simulink model "gm_uz_pu_conversion"  (R2021a)
settings: Solver=FixedStepDiscrete  StartTime=0.0  StopTime=0.02  RelTol=1e-3
undefined symbols (not defined in the file or in its folder): ampl, freq_Hz, I_B, t_ADC, V_B, v_dc
libraries: spsThreePhaseSineGeneratorLib x3
settings Model: Creator=micha  LastModifiedBy=micha
settings SolverCC: AlgebraicLoopSolver=TrustRegion
settings DataIOCC: LimitDataPoints=on  SaveOutput=off  SaveTime=off
settings OptimizationCC: BlockReduction=off  ConditionallyExecuteInputs=off  DefaultParameterBehavior=Inlined  LifeSpan=inf
settings DebuggingCC: AlgebraicLoopMsg=error  InheritedTsInSrcMsg=none  SingleTaskRateTransMsg=error  AllowSymbolicDim=off  StrictBusMsg=ErrorOnBusTreatedAsVector  SFUnexpectedBacktrackingDiag=warning  SFNoUnconditionalDefaultTransitionDiag=warning  SFExecutionAtInitializationDiag=none  SFMachineParentedDataDiag=warning  ArithmeticOperatorsInVariantConditions=warning
settings HardwareCC: ProdBitPerPointer=32  ProdBitPerSizeT=32  ProdBitPerPtrDiffT=32  ProdLargestAtomicFloat=None  ProdIntDivRoundTo=Undefined  ProdEndianess=Unspecified  ProdWordSize=32  ProdHWDeviceType=ASIC/FPGA->ASIC/FPGA  ProdEqTarget=off
settings SFSimCC: SimUseLocalCustomCode=off  CustomCodeUndefinedFunction=UseInterfaceOnly
settings RTWCC: RTWUseLocalCustomCode=off
settings CodeAppCC: StateflowObjectComments=on
settings GRTTargetCC: TargetLangStandard=C89/C90 (ANSI)
settings ConfigComp: CovScope=ReferencedModels  CovMetricSettings=dw  CovSaveCumulativeToWorkspaceVar=on  CovSaveSingleToWorkspaceVar=on  CovExternalEMLEnable=off  CovSFcnEnable=off

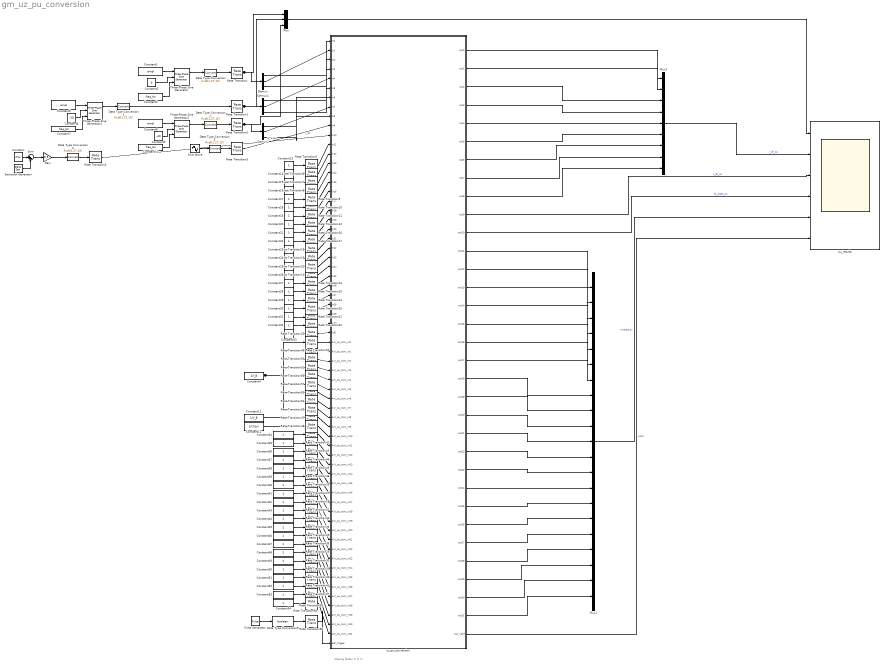
== system gm_uz_pu_conversion ==
  note: sharing factor = 0 !!!
  Constant : Constant  Value=2*pi
  Constant1 : Constant  Value=ampl
  Constant10 : Constant  Value=freq_Hz
  Constant11 : Constant  Value=1/V_B  OutDataTypeStr=fixdt(0,18,18)
  Constant12 : Constant  Value=1/(2*pi)  OutDataTypeStr=fixdt(0,18,18)
  Constant{13..33} (21 alike) : Constant  OutDataTypeStr=fixdt(1,27,15)
  Constant2 : Constant  Value=0
  Constant3 : Constant  Value=freq_Hz
  Constant{34..54} (21 alike) : Constant  OutDataTypeStr=fixdt(0,18,18)
  Constant4 : Constant  Value=1/I_B  OutDataTypeStr=fixdt(0,18,18)
  Constant5 : Constant  Value=ampl
  Constant6 : Constant  Value=-20
  Constant7 : Constant  Value=freq_Hz
  Constant8 : Constant  Value=ampl
  Constant9 : Constant  Value=-40
  Data Type Conversion{,1..4} (5 alike) : DataTypeConversion  OutDataTypeStr=fixdt(1,27,15)
  Data Type Conversion5 : DataTypeConversion  OutDataTypeStr=boolean
  Demux : Demux  Outputs=3
  Demux1 : Demux  Outputs=3
  Demux2 : Demux  Outputs=3
  Gain : Gain  Gain=0.5
  Mux : Mux  Inputs=3
  Mux1 : Mux  Inputs=21
  Mux3 : Mux  Inputs=9
  Pulse Generator : DiscretePulseGenerator  PulseType=Time based  Period=t_ADC  PulseWidth=5
  Rate Transition{,1..58} (59 alike) : RateTransition  OutPortSampleTime=ts
  Sawtooth Generator : SignalGenerator  WaveForm=sawtooth  Amplitude=2*pi  Frequency=2*pi*freq_Hz  Units=rad/sec
  Sine Wave : Sin  Amplitude=0.03*v_dc  Bias=v_dc  Frequency=2*pi*2*9*freq_Hz  SampleTime=0
  Sum : Sum  Inputs=|+-
  Three-Phase Sine Generator : spsThreePhaseSineGeneratorLib/Three-Phase Sine Generator  Ts=10e-9
      settings: SourceProductBaseCode=PS
  Three-Phase Sine Generator1 : spsThreePhaseSineGeneratorLib/Three-Phase Sine Generator  Ts=10e-9
      settings: SourceProductBaseCode=PS
  Three-Phase Sine Generator2 : spsThreePhaseSineGeneratorLib/Three-Phase Sine Generator  Ts=10e-9
      settings: SourceProductBaseCode=PS
  pu_results : Scope  NumInputPorts=6
  uz_pu_conversion : Subsystem  TreatAsAtomicUnit=on
  wires:
  uz_pu_conversion/33(out_valid) -> pu_results/6  "valid"
  Rate Transition58/1 -> uz_pu_conversion/65(adc_trigger)
  Pulse Generator/1 -> Data Type Conversion5/1
  Data Type Conversion5/1 -> Rate Transition58/1
  Mux1/1 -> pu_results/5  "unused_pu"
  uz_pu_conversion/32(out31) -> Mux1/21
  uz_pu_conversion/31(out30) -> Mux1/20
  uz_pu_conversion/30(out29) -> Mux1/19
  uz_pu_conversion/29(out28) -> Mux1/18
  uz_pu_conversion/28(out27) -> Mux1/17
  uz_pu_conversion/27(out26) -> Mux1/16
  uz_pu_conversion/26(out25) -> Mux1/15
  uz_pu_conversion/25(out24) -> Mux1/14
  uz_pu_conversion/24(out23) -> Mux1/13
  uz_pu_conversion/23(out22) -> Mux1/12
  uz_pu_conversion/22(out21) -> Mux1/11
  uz_pu_conversion/21(out20) -> Mux1/10
  uz_pu_conversion/20(out19) -> Mux1/9
  uz_pu_conversion/19(out18) -> Mux1/8
  uz_pu_conversion/18(out17) -> Mux1/7
  uz_pu_conversion/17(out16) -> Mux1/6
  uz_pu_conversion/16(out15) -> Mux1/5
  uz_pu_conversion/15(out14) -> Mux1/4
  uz_pu_conversion/14(out13) -> Mux1/3
  uz_pu_conversion/13(out12) -> Mux1/2
  uz_pu_conversion/12(out11) -> Mux1/1
  Constant52/1 -> Rate Transition37/1
  Constant51/1 -> Rate Transition41/1
  Constant50/1 -> Rate Transition40/1
  Constant54/1 -> Rate Transition39/1
  Constant53/1 -> Rate Transition38/1
  Constant42/1 -> Rate Transition32/1
  Constant43/1 -> Rate Transition33/1
  Constant44/1 -> Rate Transition34/1
  Constant48/1 -> Rate Transition30/1
  Constant45/1 -> Rate Transition35/1
  Constant49/1 -> Rate Transition31/1
  Constant46/1 -> Rate Transition36/1
  Constant47/1 -> Rate Transition29/1
  Constant38/1 -> Rate Transition46/1
  Constant39/1 -> Rate Transition26/1
  Constant40/1 -> Rate Transition27/1
  Constant41/1 -> Rate Transition28/1
  Constant36/1 -> Rate Transition44/1
  Constant37/1 -> Rate Transition45/1
  Constant35/1 -> Rate Transition43/1
  Constant34/1 -> Rate Transition42/1
  Constant33/1 -> Rate Transition23/1
  Constant31/1 -> Rate Transition21/1
  Constant32/1 -> Rate Transition22/1
  Constant29/1 -> Rate Transition24/1
  Constant30/1 -> Rate Transition25/1
  Constant28/1 -> Rate Transition15/1
  Constant27/1 -> Rate Transition14/1
  Constant25/1 -> Rate Transition20/1
  Constant26/1 -> Rate Transition13/1
  Constant24/1 -> Rate Transition19/1
  Constant23/1 -> Rate Transition18/1
  Constant21/1 -> Rate Transition16/1
  Constant22/1 -> Rate Transition17/1
  Constant20/1 -> Rate Transition12/1
  Constant19/1 -> Rate Transition11/1
  Constant17/1 -> Rate Transition9/1
  Constant18/1 -> Rate Transition10/1
  Constant16/1 -> Rate Transition8/1
  Constant15/1 -> Rate Transition7/1
  Constant14/1 -> Rate Transition6/1
  Constant13/1 -> Rate Transition5/1
  Rate Transition1/1 -> Demux1/1, Mux/2
  Mux/1 -> pu_results/1
  Rate Transition56/1 -> uz_pu_conversion/37(AXI_pu_conv_in4)
  Rate Transition57/1 -> uz_pu_conversion/38(AXI_pu_conv_in5)
  Rate Transition55/1 -> uz_pu_conversion/41(AXI_pu_conv_in8)
  Rate Transition54/1 -> uz_pu_conversion/40(AXI_pu_conv_in7)
  Rate Transition51/1 -> uz_pu_conversion/36(AXI_pu_conv_in3)
  Rate Transition52/1 -> uz_pu_conversion/33(AXI_pu_conv_in0)
  Rate Transition53/1 -> uz_pu_conversion/39(AXI_pu_conv_in6)
  Rate Transition49/1 -> uz_pu_conversion/34(AXI_pu_conv_in1)
  Rate Transition50/1 -> uz_pu_conversion/35(AXI_pu_conv_in2)
  Rate Transition48/1 -> uz_pu_conversion/43(AXI_pu_conv_in10)
  Rate Transition47/1 -> uz_pu_conversion/42(AXI_pu_conv_in9)
  Rate Transition42/1 -> uz_pu_conversion/44(AXI_pu_conv_in11)
  Rate Transition33/1 -> uz_pu_conversion/53(AXI_pu_conv_in20)
  Rate Transition29/1 -> uz_pu_conversion/57(AXI_pu_conv_in24)
  Rate Transition46/1 -> uz_pu_conversion/48(AXI_pu_conv_in15)
  Rate Transition35/1 -> uz_pu_conversion/55(AXI_pu_conv_in22)
  Rate Transition28/1 -> uz_pu_conversion/51(AXI_pu_conv_in18)
  Rate Transition44/1 -> uz_pu_conversion/46(AXI_pu_conv_in13)
  Rate Transition45/1 -> uz_pu_conversion/47(AXI_pu_conv_in14)
  Rate Transition40/1 -> uz_pu_conversion/60(AXI_pu_conv_in27)
  Rate Transition26/1 -> uz_pu_conversion/49(AXI_pu_conv_in16)
  Rate Transition27/1 -> uz_pu_conversion/50(AXI_pu_conv_in17)
  Rate Transition37/1 -> uz_pu_conversion/62(AXI_pu_conv_in29)
  Rate Transition30/1 -> uz_pu_conversion/58(AXI_pu_conv_in25)
  Rate Transition38/1 -> uz_pu_conversion/63(AXI_pu_conv_in30)
  Rate Transition41/1 -> uz_pu_conversion/61(AXI_pu_conv_in28)
  Rate Transition39/1 -> uz_pu_conversion/64(AXI_pu_conv_in31)
  Rate Transition43/1 -> uz_pu_conversion/45(AXI_pu_conv_in12)
  Rate Transition31/1 -> uz_pu_conversion/59(AXI_pu_conv_in26)
  Rate Transition36/1 -> uz_pu_conversion/56(AXI_pu_conv_in23)
  Rate Transition32/1 -> uz_pu_conversion/52(AXI_pu_conv_in19)
  Rate Transition34/1 -> uz_pu_conversion/54(AXI_pu_conv_in21)
  Rate Transition21/1 -> uz_pu_conversion/30(in29)
  Rate Transition24/1 -> uz_pu_conversion/28(in27)
  Rate Transition25/1 -> uz_pu_conversion/29(in28)
  Rate Transition22/1 -> uz_pu_conversion/31(in30)
  Rate Transition23/1 -> uz_pu_conversion/32(in31)
  Rate Transition14/1 -> uz_pu_conversion/26(in25)
  Rate Transition15/1 -> uz_pu_conversion/27(in26)
  Rate Transition20/1 -> uz_pu_conversion/24(in23)
  Rate Transition18/1 -> uz_pu_conversion/22(in21)
  Rate Transition19/1 -> uz_pu_conversion/23(in22)
  Rate Transition17/1 -> uz_pu_conversion/21(in20)
  Rate Transition16/1 -> uz_pu_conversion/20(in19)
  Rate Transition13/1 -> uz_pu_conversion/25(in24)
  Rate Transition11/1 -> uz_pu_conversion/18(in17)
  Rate Transition12/1 -> uz_pu_conversion/19(in18)
  Rate Transition10/1 -> uz_pu_conversion/17(in16)
  Rate Transition9/1 -> uz_pu_conversion/16(in15)
  Rate Transition8/1 -> uz_pu_conversion/15(in14)
  Rate Transition7/1 -> uz_pu_conversion/14(in13)
  Rate Transition6/1 -> uz_pu_conversion/13(in12)
  Rate Transition5/1 -> uz_pu_conversion/12(in11)
  Sum/1 -> Gain/1
  Gain/1 -> Data Type Conversion4/1
  Constant/1 -> Sum/1
  uz_pu_conversion/11(out10) -> pu_results/4  "el_angle_pu"
  Constant12/1 -> Rate Transition48/1
  Sawtooth Generator/1 -> Sum/2
  Rate Transition4/1 -> uz_pu_conversion/11(in10)  "el_angle"
  Data Type Conversion4/1 -> Rate Transition4/1
  Data Type Conversion3/1 -> Rate Transition3/1
  uz_pu_conversion/10(out9) -> pu_results/3  "v_dc_pu"
  Sine Wave/1 -> Data Type Conversion3/1
  Rate Transition3/1 -> uz_pu_conversion/10(in9)  "v_dc"
  Constant11/1 -> Rate Transition47/1
  uz_pu_conversion/9(out8) -> Mux3/9
  uz_pu_conversion/8(out7) -> Mux3/8
  uz_pu_conversion/7(out6) -> Mux3/7
  Demux2/3 -> uz_pu_conversion/9(in8)
  Demux2/2 -> uz_pu_conversion/8(in7)
  Demux2/1 -> uz_pu_conversion/7(in6)
  Rate Transition2/1 -> Demux2/1, Mux/3
  Constant10/1 -> Three-Phase Sine Generator2/3
  Constant9/1 -> Three-Phase Sine Generator2/2
  Three-Phase Sine Generator2/1 -> Data Type Conversion2/1
  Constant8/1 -> Three-Phase Sine Generator2/1
  Data Type Conversion2/1 -> Rate Transition2/1
  Demux1/3 -> uz_pu_conversion/6(in5)
  Demux1/2 -> uz_pu_conversion/5(in4)
  Demux1/1 -> uz_pu_conversion/4(in3)
  Mux3/1 -> pu_results/2  "i_ph_pu"
  uz_pu_conversion/4(out3) -> Mux3/4
  uz_pu_conversion/3(out2) -> Mux3/3
  uz_pu_conversion/2(out1) -> Mux3/2
  uz_pu_conversion/1(out0) -> Mux3/1
  uz_pu_conversion/5(out4) -> Mux3/5
  uz_pu_conversion/6(out5) -> Mux3/6
  Constant4/1 -> Rate Transition55/1, Rate Transition54/1, Rate Transition53/1, Rate Transition57/1, Rate Transition51/1, Rate Transition50/1, Rate Transition49/1, Rate Transition52/1, Rate Transition56/1
  Three-Phase Sine Generator1/1 -> Data Type Conversion1/1
  Constant5/1 -> Three-Phase Sine Generator1/1
  Data Type Conversion1/1 -> Rate Transition1/1
  Constant7/1 -> Three-Phase Sine Generator1/3
  Constant6/1 -> Three-Phase Sine Generator1/2
  Demux/3 -> uz_pu_conversion/3(in2)
  Demux/2 -> uz_pu_conversion/2(in1)
  Data Type Conversion/1 -> Rate Transition/1
  Demux/1 -> uz_pu_conversion/1(in0)
  Rate Transition/1 -> Mux/1, Demux/1
  Constant3/1 -> Three-Phase Sine Generator/3
  Constant2/1 -> Three-Phase Sine Generator/2
  Constant1/1 -> Three-Phase Sine Generator/1
  Three-Phase Sine Generator/1 -> Data Type Conversion/1

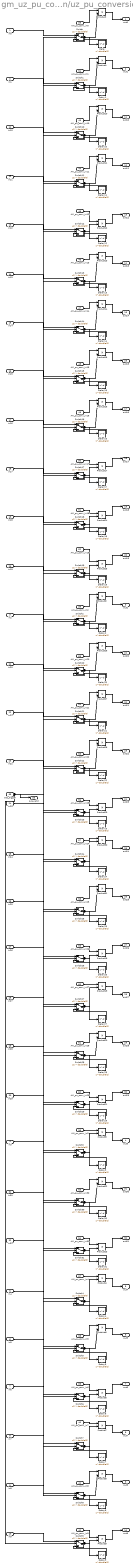
== system gm_uz_pu_conversion/uz_pu_conversion ==
  in0 : Inport  OutDataTypeStr=fixdt(1, 27, 15)  PortDimensions=1  SampleTime=1e-08
  in1 : Inport  Port=2  OutDataTypeStr=fixdt(1, 27, 15)  PortDimensions=1  SampleTime=1e-08
  in2 : Inport  Port=3  OutDataTypeStr=fixdt(1, 27, 15)  PortDimensions=1  SampleTime=1e-08
  in3 : Inport  Port=4  OutDataTypeStr=fixdt(1, 27, 15)  PortDimensions=1  SampleTime=1e-08
  in4 : Inport  Port=5  OutDataTypeStr=fixdt(1, 27, 15)  PortDimensions=1  SampleTime=1e-08
  in5 : Inport  Port=6  OutDataTypeStr=fixdt(1, 27, 15)  PortDimensions=1  SampleTime=1e-08
  in6 : Inport  Port=7  OutDataTypeStr=fixdt(1, 27, 15)  PortDimensions=1  SampleTime=1e-08
  in7 : Inport  Port=8  OutDataTypeStr=fixdt(1, 27, 15)  PortDimensions=1  SampleTime=1e-08
  in8 : Inport  Port=9  OutDataTypeStr=fixdt(1, 27, 15)  PortDimensions=1  SampleTime=1e-08
  in9 : Inport  Port=10  OutDataTypeStr=fixdt(1, 27, 15)  PortDimensions=1  SampleTime=1e-08
  in10 : Inport  Port=11  OutDataTypeStr=fixdt(1, 27, 15)  PortDimensions=1  SampleTime=1e-08
  in11 : Inport  Port=12  OutDataTypeStr=fixdt(1, 27, 15)  PortDimensions=1  SampleTime=1e-08
  in12 : Inport  Port=13  OutDataTypeStr=fixdt(1, 27, 15)  PortDimensions=1  SampleTime=1e-08
  in13 : Inport  Port=14  OutDataTypeStr=fixdt(1, 27, 15)  PortDimensions=1  SampleTime=1e-08
  in14 : Inport  Port=15  OutDataTypeStr=fixdt(1, 27, 15)  PortDimensions=1  SampleTime=1e-08
  in15 : Inport  Port=16  OutDataTypeStr=fixdt(1, 27, 15)  PortDimensions=1  SampleTime=1e-08
  in16 : Inport  Port=17  OutDataTypeStr=fixdt(1, 27, 15)  PortDimensions=1  SampleTime=1e-08
  in17 : Inport  Port=18  OutDataTypeStr=fixdt(1, 27, 15)  PortDimensions=1  SampleTime=1e-08
  in18 : Inport  Port=19  OutDataTypeStr=fixdt(1, 27, 15)  PortDimensions=1  SampleTime=1e-08
  in19 : Inport  Port=20  OutDataTypeStr=fixdt(1, 27, 15)  PortDimensions=1  SampleTime=1e-08
  in20 : Inport  Port=21  OutDataTypeStr=fixdt(1, 27, 15)  PortDimensions=1  SampleTime=1e-08
  in21 : Inport  Port=22  OutDataTypeStr=fixdt(1, 27, 15)  PortDimensions=1  SampleTime=1e-08
  in22 : Inport  Port=23  OutDataTypeStr=fixdt(1, 27, 15)  PortDimensions=1  SampleTime=1e-08
  in23 : Inport  Port=24  OutDataTypeStr=fixdt(1, 27, 15)  PortDimensions=1  SampleTime=1e-08
  in24 : Inport  Port=25  OutDataTypeStr=fixdt(1, 27, 15)  PortDimensions=1  SampleTime=1e-08
  in25 : Inport  Port=26  OutDataTypeStr=fixdt(1, 27, 15)  PortDimensions=1  SampleTime=1e-08
  in26 : Inport  Port=27  OutDataTypeStr=fixdt(1, 27, 15)  PortDimensions=1  SampleTime=1e-08
  in27 : Inport  Port=28  OutDataTypeStr=fixdt(1, 27, 15)  PortDimensions=1  SampleTime=1e-08
  in28 : Inport  Port=29  OutDataTypeStr=fixdt(1, 27, 15)  PortDimensions=1  SampleTime=1e-08
  in29 : Inport  Port=30  OutDataTypeStr=fixdt(1, 27, 15)  PortDimensions=1  SampleTime=1e-08
  in30 : Inport  Port=31  OutDataTypeStr=fixdt(1, 27, 15)  PortDimensions=1  SampleTime=1e-08
  in31 : Inport  Port=32  OutDataTypeStr=fixdt(1, 27, 15)  PortDimensions=1  SampleTime=1e-08
  AXI_pu_conv_in0 : Inport  Port=33  OutDataTypeStr=fixdt(0, 18, 18)  PortDimensions=1  SampleTime=1e-08
  AXI_pu_conv_in1 : Inport  Port=34  OutDataTypeStr=fixdt(0, 18, 18)  PortDimensions=1  SampleTime=1e-08
  AXI_pu_conv_in2 : Inport  Port=35  OutDataTypeStr=fixdt(0, 18, 18)  PortDimensions=1  SampleTime=1e-08
  AXI_pu_conv_in3 : Inport  Port=36  OutDataTypeStr=fixdt(0, 18, 18)  PortDimensions=1  SampleTime=1e-08
  AXI_pu_conv_in4 : Inport  Port=37  OutDataTypeStr=fixdt(0, 18, 18)  PortDimensions=1  SampleTime=1e-08
  AXI_pu_conv_in5 : Inport  Port=38  OutDataTypeStr=fixdt(0, 18, 18)  PortDimensions=1  SampleTime=1e-08
  AXI_pu_conv_in6 : Inport  Port=39  OutDataTypeStr=fixdt(0, 18, 18)  PortDimensions=1  SampleTime=1e-08
  AXI_pu_conv_in7 : Inport  Port=40  OutDataTypeStr=fixdt(0, 18, 18)  PortDimensions=1  SampleTime=1e-08
  AXI_pu_conv_in8 : Inport  Port=41  OutDataTypeStr=fixdt(0, 18, 18)  PortDimensions=1  SampleTime=1e-08
  AXI_pu_conv_in9 : Inport  Port=42  OutDataTypeStr=fixdt(0, 18, 18)  PortDimensions=1  SampleTime=1e-08
  AXI_pu_conv_in10 : Inport  Port=43  OutDataTypeStr=fixdt(0, 18, 18)  PortDimensions=1  SampleTime=1e-08
  AXI_pu_conv_in11 : Inport  Port=44  OutDataTypeStr=fixdt(0, 18, 18)  PortDimensions=1  SampleTime=1e-08
  AXI_pu_conv_in12 : Inport  Port=45  OutDataTypeStr=fixdt(0, 18, 18)  PortDimensions=1  SampleTime=1e-08
  AXI_pu_conv_in13 : Inport  Port=46  OutDataTypeStr=fixdt(0, 18, 18)  PortDimensions=1  SampleTime=1e-08
  AXI_pu_conv_in14 : Inport  Port=47  OutDataTypeStr=fixdt(0, 18, 18)  PortDimensions=1  SampleTime=1e-08
  AXI_pu_conv_in15 : Inport  Port=48  OutDataTypeStr=fixdt(0, 18, 18)  PortDimensions=1  SampleTime=1e-08
  AXI_pu_conv_in16 : Inport  Port=49  OutDataTypeStr=fixdt(0, 18, 18)  PortDimensions=1  SampleTime=1e-08
  AXI_pu_conv_in17 : Inport  Port=50  OutDataTypeStr=fixdt(0, 18, 18)  PortDimensions=1  SampleTime=1e-08
  AXI_pu_conv_in18 : Inport  Port=51  OutDataTypeStr=fixdt(0, 18, 18)  PortDimensions=1  SampleTime=1e-08
  AXI_pu_conv_in19 : Inport  Port=52  OutDataTypeStr=fixdt(0, 18, 18)  PortDimensions=1  SampleTime=1e-08
  AXI_pu_conv_in20 : Inport  Port=53  OutDataTypeStr=fixdt(0, 18, 18)  PortDimensions=1  SampleTime=1e-08
  AXI_pu_conv_in21 : Inport  Port=54  OutDataTypeStr=fixdt(0, 18, 18)  PortDimensions=1  SampleTime=1e-08
  AXI_pu_conv_in22 : Inport  Port=55  OutDataTypeStr=fixdt(0, 18, 18)  PortDimensions=1  SampleTime=1e-08
  AXI_pu_conv_in23 : Inport  Port=56  OutDataTypeStr=fixdt(0, 18, 18)  PortDimensions=1  SampleTime=1e-08
  AXI_pu_conv_in24 : Inport  Port=57  OutDataTypeStr=fixdt(0, 18, 18)  PortDimensions=1  SampleTime=1e-08
  AXI_pu_conv_in25 : Inport  Port=58  OutDataTypeStr=fixdt(0, 18, 18)  PortDimensions=1  SampleTime=1e-08
  AXI_pu_conv_in26 : Inport  Port=59  OutDataTypeStr=fixdt(0, 18, 18)  PortDimensions=1  SampleTime=1e-08
  AXI_pu_conv_in27 : Inport  Port=60  OutDataTypeStr=fixdt(0, 18, 18)  PortDimensions=1  SampleTime=1e-08
  AXI_pu_conv_in28 : Inport  Port=61  OutDataTypeStr=fixdt(0, 18, 18)  PortDimensions=1  SampleTime=1e-08
  AXI_pu_conv_in29 : Inport  Port=62  OutDataTypeStr=fixdt(0, 18, 18)  PortDimensions=1  SampleTime=1e-08
  AXI_pu_conv_in30 : Inport  Port=63  OutDataTypeStr=fixdt(0, 18, 18)  PortDimensions=1  SampleTime=1e-08
  AXI_pu_conv_in31 : Inport  Port=64  OutDataTypeStr=fixdt(0, 18, 18)  PortDimensions=1  SampleTime=1e-08
  adc_trigger : Inport  Port=65  OutDataTypeStr=boolean  PortDimensions=1  SampleTime=1e-08
  Delay{,1..31} (32 alike) : Delay  DelayLength=double(1)  InitialCondition=0  SampleTime=1e-08
  Product{,1..31} (32 alike) : Product  Inputs=**  OutDataTypeStr=fixdt(1, 18, 15)  SampleTime=1e-08
  Switch{,1..31} (32 alike) : Switch  Criteria=u2 > Threshold  Threshold=double(0)  OutDataTypeStr=fixdt(1, 27, 15)  SampleTime=1e-08
  out0 : Outport  SampleTime=1e-08
  out1 : Outport  Port=2  SampleTime=1e-08
  out2 : Outport  Port=3  SampleTime=1e-08
  out3 : Outport  Port=4  SampleTime=1e-08
  out4 : Outport  Port=5  SampleTime=1e-08
  out5 : Outport  Port=6  SampleTime=1e-08
  out6 : Outport  Port=7  SampleTime=1e-08
  out7 : Outport  Port=8  SampleTime=1e-08
  out8 : Outport  Port=9  SampleTime=1e-08
  out9 : Outport  Port=10  SampleTime=1e-08
  out10 : Outport  Port=11  SampleTime=1e-08
  out11 : Outport  Port=12  SampleTime=1e-08
  out12 : Outport  Port=13  SampleTime=1e-08
  out13 : Outport  Port=14  SampleTime=1e-08
  out14 : Outport  Port=15  SampleTime=1e-08
  out15 : Outport  Port=16  SampleTime=1e-08
  out16 : Outport  Port=17  SampleTime=1e-08
  out17 : Outport  Port=18  SampleTime=1e-08
  out18 : Outport  Port=19  SampleTime=1e-08
  out19 : Outport  Port=20  SampleTime=1e-08
  out20 : Outport  Port=21  SampleTime=1e-08
  out21 : Outport  Port=22  SampleTime=1e-08
  out22 : Outport  Port=23  SampleTime=1e-08
  out23 : Outport  Port=24  SampleTime=1e-08
  out24 : Outport  Port=25  SampleTime=1e-08
  out25 : Outport  Port=26  SampleTime=1e-08
  out26 : Outport  Port=27  SampleTime=1e-08
  out27 : Outport  Port=28  SampleTime=1e-08
  out28 : Outport  Port=29  SampleTime=1e-08
  out29 : Outport  Port=30  SampleTime=1e-08
  out30 : Outport  Port=31  SampleTime=1e-08
  out31 : Outport  Port=32  SampleTime=1e-08
  out_valid : Outport  Port=33  OutDataTypeStr=boolean  SampleTime=1e-08  LockScale=on
  wires:
  in0/1 -> Switch/1
  in1/1 -> Switch1/1
  in2/1 -> Switch2/1
  in3/1 -> Switch3/1
  in4/1 -> Switch4/1
  in5/1 -> Switch5/1
  in6/1 -> Switch6/1
  in7/1 -> Switch7/1
  in8/1 -> Switch8/1
  in9/1 -> Switch9/1
  in10/1 -> Switch10/1
  in11/1 -> Switch11/1
  in12/1 -> Switch12/1
  in13/1 -> Switch13/1
  in14/1 -> Switch14/1
  in15/1 -> Switch15/1
  in16/1 -> Switch16/1
  in17/1 -> Switch17/1
  in18/1 -> Switch18/1
  in19/1 -> Switch19/1
  in20/1 -> Switch20/1
  in21/1 -> Switch21/1
  in22/1 -> Switch22/1
  in23/1 -> Switch23/1
  in24/1 -> Switch24/1
  in25/1 -> Switch25/1
  in26/1 -> Switch26/1
  in27/1 -> Switch27/1
  in28/1 -> Switch28/1
  in29/1 -> Switch29/1
  in30/1 -> Switch30/1
  in31/1 -> Switch31/1
  AXI_pu_conv_in0/1 -> Product/1
  AXI_pu_conv_in1/1 -> Product1/1
  AXI_pu_conv_in2/1 -> Product2/1
  AXI_pu_conv_in3/1 -> Product3/1
  AXI_pu_conv_in4/1 -> Product4/1
  AXI_pu_conv_in5/1 -> Product5/1
  AXI_pu_conv_in6/1 -> Product6/1
  AXI_pu_conv_in7/1 -> Product7/1
  AXI_pu_conv_in8/1 -> Product8/1
  AXI_pu_conv_in9/1 -> Product9/1
  AXI_pu_conv_in10/1 -> Product10/1
  AXI_pu_conv_in11/1 -> Product11/1
  AXI_pu_conv_in12/1 -> Product12/1
  AXI_pu_conv_in13/1 -> Product13/1
  AXI_pu_conv_in14/1 -> Product14/1
  AXI_pu_conv_in15/1 -> Product15/1
  AXI_pu_conv_in16/1 -> Product16/1
  AXI_pu_conv_in17/1 -> Product17/1
  AXI_pu_conv_in18/1 -> Product24/1
  AXI_pu_conv_in19/1 -> Product25/1
  AXI_pu_conv_in20/1 -> Product26/1
  AXI_pu_conv_in21/1 -> Product27/1
  AXI_pu_conv_in22/1 -> Product28/1
  AXI_pu_conv_in23/1 -> Product29/1
  AXI_pu_conv_in24/1 -> Product30/1
  AXI_pu_conv_in25/1 -> Product31/1
  AXI_pu_conv_in26/1 -> Product18/1
  AXI_pu_conv_in27/1 -> Product19/1
  AXI_pu_conv_in28/1 -> Product20/1
  AXI_pu_conv_in29/1 -> Product21/1
  AXI_pu_conv_in30/1 -> Product22/1
  AXI_pu_conv_in31/1 -> Product23/1
  adc_trigger/1 -> Switch9/2, Switch8/2, Switch7/2, Switch6/2, Switch5/2, Switch4/2, Switch31/2, Switch30/2, Switch3/2, Switch29/2, Switch28/2, Switch27/2, Switch26/2, Switch25/2, Switch24/2, Switch23/2, Switch22/2, Switch21/2, Switch20/2, Switch2/2, Switch19/2, Switch18/2, Switch17/2, Switch16/2, Switch15/2, Switch14/2, Switch13/2, Switch12/2, Switch11/2, Switch10/2, Switch1/2, Switch/2, out_valid/1
  Delay/1 -> Switch/3
  Delay1/1 -> Switch1/3
  Delay10/1 -> Switch10/3
  Delay11/1 -> Switch11/3
  Delay12/1 -> Switch12/3
  Delay13/1 -> Switch13/3
  Delay14/1 -> Switch14/3
  Delay15/1 -> Switch15/3
  Delay16/1 -> Switch16/3
  Delay17/1 -> Switch17/3
  Delay18/1 -> Switch18/3
  Delay19/1 -> Switch19/3
  Delay2/1 -> Switch2/3
  Delay20/1 -> Switch20/3
  Delay21/1 -> Switch21/3
  Delay22/1 -> Switch22/3
  Delay23/1 -> Switch23/3
  Delay24/1 -> Switch24/3
  Delay25/1 -> Switch25/3
  Delay26/1 -> Switch26/3
  Delay27/1 -> Switch27/3
  Delay28/1 -> Switch28/3
  Delay29/1 -> Switch29/3
  Delay3/1 -> Switch3/3
  Delay30/1 -> Switch30/3
  Delay31/1 -> Switch31/3
  Delay4/1 -> Switch4/3
  Delay5/1 -> Switch5/3
  Delay6/1 -> Switch6/3
  Delay7/1 -> Switch7/3
  Delay8/1 -> Switch8/3
  Delay9/1 -> Switch9/3
  Product/1 -> out0/1
  Product1/1 -> out1/1
  Product10/1 -> out10/1
  Product11/1 -> out11/1
  Product12/1 -> out12/1
  Product13/1 -> out13/1
  Product14/1 -> out14/1
  Product15/1 -> out15/1
  Product16/1 -> out16/1
  Product17/1 -> out17/1
  Product18/1 -> out26/1
  Product19/1 -> out27/1
  Product2/1 -> out2/1
  Product20/1 -> out28/1
  Product21/1 -> out29/1
  Product22/1 -> out30/1
  Product23/1 -> out31/1
  Product24/1 -> out18/1
  Product25/1 -> out19/1
  Product26/1 -> out20/1
  Product27/1 -> out21/1
  Product28/1 -> out22/1
  Product29/1 -> out23/1
  Product3/1 -> out3/1
  Product30/1 -> out24/1
  Product31/1 -> out25/1
  Product4/1 -> out4/1
  Product5/1 -> out5/1
  Product6/1 -> out6/1
  Product7/1 -> out7/1
  Product8/1 -> out8/1
  Product9/1 -> out9/1
  Switch/1 -> Product/2, Delay/1
  Switch1/1 -> Product1/2, Delay1/1
  Switch10/1 -> Product10/2, Delay10/1
  Switch11/1 -> Product11/2, Delay11/1
  Switch12/1 -> Product12/2, Delay12/1
  Switch13/1 -> Product13/2, Delay13/1
  Switch14/1 -> Product14/2, Delay14/1
  Switch15/1 -> Product15/2, Delay15/1
  Switch16/1 -> Product16/2, Delay16/1
  Switch17/1 -> Product17/2, Delay17/1
  Switch18/1 -> Product24/2, Delay18/1
  Switch19/1 -> Product25/2, Delay19/1
  Switch2/1 -> Product2/2, Delay2/1
  Switch20/1 -> Product26/2, Delay20/1
  Switch21/1 -> Product27/2, Delay21/1
  Switch22/1 -> Product28/2, Delay22/1
  Switch23/1 -> Product29/2, Delay23/1
  Switch24/1 -> Product30/2, Delay24/1
  Switch25/1 -> Product31/2, Delay25/1
  Switch26/1 -> Product18/2, Delay26/1
  Switch27/1 -> Product19/2, Delay27/1
  Switch28/1 -> Product20/2, Delay28/1
  Switch29/1 -> Product21/2, Delay29/1
  Switch3/1 -> Product3/2, Delay3/1
  Switch30/1 -> Product22/2, Delay30/1
  Switch31/1 -> Product23/2, Delay31/1
  Switch4/1 -> Product4/2, Delay4/1
  Switch5/1 -> Product5/2, Delay5/1
  Switch6/1 -> Product6/2, Delay6/1
  Switch7/1 -> Product7/2, Delay7/1
  Switch8/1 -> Product8/2, Delay8/1
  Switch9/1 -> Product9/2, Delay9/1
